simulink model "Lock_Control_Vy"  (Simulink 7.9)
settings: Solver=FixedStepDiscrete  StartTime=0.0  StopTime=0.8  RelTol=1e-3  SampleTimeConstraint=STIndependent
PreLoadFcn:
  | Locking_Strategy_selfinit
values from neighbouring files (symbols this model uses):
  lockDoor_speedThreshTimer = mpt.Parameter    [Locking_Strategy_selfinit.m]
  lockDoor_speedThreshValue = mpt.Parameter    [Locking_Strategy_selfinit.m]
libraries: common_lib x1
CloseFcn:
  | rtwprivate ssgencode ModelCloseRequest ADL
settings Model: MinMaxOverflowLogging=ForceOff  Creator=fguerin  LastModifiedBy=klindqvi  CovMetricSettings=dcme  CovHtmlReporting=off  covSaveCumulativeToWorkspaceVar=off  CovSaveSingleToWorkspaceVar=off  CovModelRefEnable=off  CovExternalEMLEnable=on
settings DataIOCC: ExternalInput=[t,u]  LimitDataPoints=off  LoadExternalInput=on  SaveOutput=off  DSMLogging=off  SaveTime=off  SignalLoggingName=logsOut
settings OptimizationCC: InlineParams=on  InlineInvariantSignals=on  EnhancedBackFolding=on  ZeroExternalMemoryAtStartup=off  ZeroInternalMemoryAtStartup=off  EfficientFloat2IntCast=on  OptimizeModelRefInitCode=on  LifeSpan=1
settings DebuggingCC: ReadBeforeWriteMsg=EnableAllAsError  WriteAfterWriteMsg=EnableAllAsError  WriteAfterReadMsg=EnableAllAsError  AlgebraicLoopMsg=error  ArtificialAlgebraicLoopMsg=error  SaveWithDisabledLinksMsg=error  SaveWithParameterizedLinksMsg=error  CheckExecutionContextPreStartOutputMsg=on  CheckExecutionContextRuntimeOutputMsg=on  BlockPriorityViolationMsg=error  SolverPrmCheckMsg=error  MultiTaskCondExecSysMsg=warning  MultiTaskRateTransMsg=warning  IntegerOverflowMsg=none  ParameterUnderflowMsg=error  ParameterPrecisionLossMsg=error  ParameterTunabilityLossMsg=error  UnderSpecifiedDataTypeMsg=warning  UnnecessaryDatatypeConvMsg=warning  VectorMatrixConversionMsg=error  SignalLabelMismatchMsg=warning  SFcnCompatibilityMsg=error  BusObjectLabelMismatch=error  RootOutportRequireBusObject=error  AssertControl=DisableAll  ModelReferenceIOMsg=error  ModelReferenceIOMismatchMessage=error  ModelReferenceCSMismatchMessage=warning  UnknownTsInhSupMsg=error  ModelReferenceDataLoggingMessage=error  ModelReferenceSymbolNameMessage=none  StrictBusMsg=ErrorOnBusTreatedAsVector
settings HardwareCC: ProdLargestAtomicInteger=Long  ProdLargestAtomicFloat=Double  ProdIntDivRoundTo=Zero  ProdEndianess=BigEndian  ProdHWDeviceType=Freescale->MPC5500
settings ModelReferenceCC: ModelReferenceNumInstancesAllowed=Single
settings SFSimCC: SimParseCustomCode=off
settings RTWCC: SystemTargetFile=ert.tlc  TemplateMakefile=ert_default_tmf  Description=Embedded Coder  GenerateReport=on  RTWVerbose=off  ProcessScript=ert_make_rtw_hook  IncludeHyperlinkInReport=on  LaunchReport=on  GenerateTraceInfo=on  GenerateTraceReport=on  GenerateTraceReportSl=on  GenerateTraceReportSf=on  GenerateTraceReportEml=on  GenerateCodeMetricsReport=on
settings MATStruct: className=rtw.pil.Bullseye  argsAllComponents=[]  excludedModels=[]  includeReferencedModels=off  includeTopModel=on  enabled=on
settings CodeAppCC: ForceParamTrailComments=on  IgnoreCustomStorageClasses=off  IgnoreTestpoints=on  MangleLength=4  InlinedPrmAccess=Macros  ReqsInCode=on
settings ERTTargetCC: CodeReplacementLibrary=ANSI_C  MultiwordLength=2048  SupportAbsoluteTime=off  SupportNonFinite=off  SupportComplex=off  PortableWordSizes=on  InlinedParameterPlacement=NonHierarchical  ERTCustomFileTemplate=example_file_process.tlc  ConvertIfToSwitch=off  SuppressUnreachableDefaultCases=off
settings ConfigComp: Description=Design Verifier Custom Configuration Component  DVMaxProcessTime=600  DVDisplayUnsatisfiableObjectives=on  DVAutomaticStubbing=off  DVOutputDir=C:\Work\Data\Pilots\P_PSA_ECoder_BenchMark_LaGarenne\source9b\deliverable\trunk\demos\VnV_example\Projects\ADL_Project/Simulink_Test_Generation/ADL_Sim  DVModelCoverageObjectives=MCDC  DVTestSuiteOptimization=CombinedObjectives  DVDataFileName=./Tests/$ModelName$_sldvdata  DVSaveHarnessModel=on  DVHarnessModelFileName=./Tests/$ModelName$_testHarness  DVModelReferenceHarness=on  DVSaveReport=on  DVReportFileName=ADL_Sim_SLDV.html

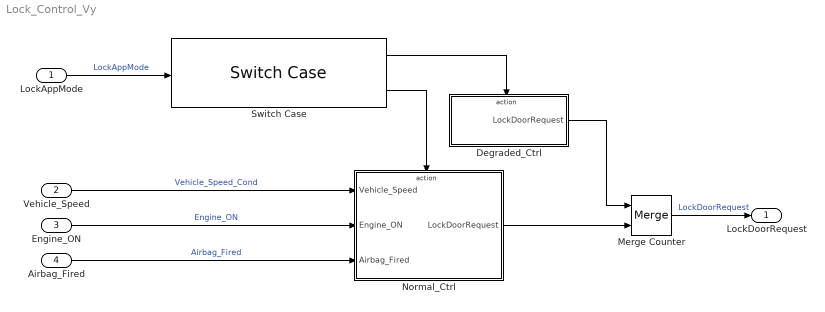
== system Lock_Control_Vy ==
  LockAppMode : Inport  PortDimensions=1
  Vehicle_Speed : Inport  Port=2  OutDataTypeStr=single  PortDimensions=1
  Engine_ON : Inport  Port=3  OutDataTypeStr=boolean  PortDimensions=1
  Airbag_Fired : Inport  Port=4  OutDataTypeStr=boolean  PortDimensions=1
  Degraded_Ctrl : Subsystem
  Merge Counter : Merge
  Normal_Ctrl : Subsystem
  Switch Case : SwitchCase  CaseConditions={LockingMode.FAILURE,[LockingMode.NORMAL_UNLOCK,LockingMode.NORMAL_LOCK]}  ShowDefaultCase=off
  LockDoorRequest : Outport  OutDataTypeStr=boolean  PortDimensions=1
  wires:
  LockAppMode/1 -> Switch Case/1  "LockAppMode"
  Vehicle_Speed/1 -> Normal_Ctrl/1(Vehicle_Speed)  "Vehicle_Speed_Cond"
  Engine_ON/1 -> Normal_Ctrl/2(Engine_ON)  "Engine_ON"
  Degraded_Ctrl/1(LockDoorRequest) -> Merge Counter/1
  Normal_Ctrl/1(LockDoorRequest) -> Merge Counter/2
  Merge Counter/1 -> LockDoorRequest/1  "LockDoorRequest"
  Switch Case/1 -> Degraded_Ctrl/Action
  Switch Case/2 -> Normal_Ctrl/Action
  Airbag_Fired/1 -> Normal_Ctrl/3(Airbag_Fired)  "Airbag_Fired"

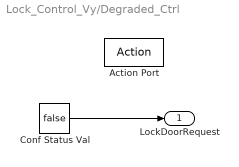
== system Lock_Control_Vy/Degraded_Ctrl ==
  Action Port : ActionPort  ActionType=case
  Conf Status Val : Constant  Value=false  OutDataTypeStr=Inherit: Inherit via back propagation  SampleTime=-1
  LockDoorRequest : Outport  OutDataTypeStr=boolean  PortDimensions=1
  wires:
  Conf Status Val/1 -> LockDoorRequest/1

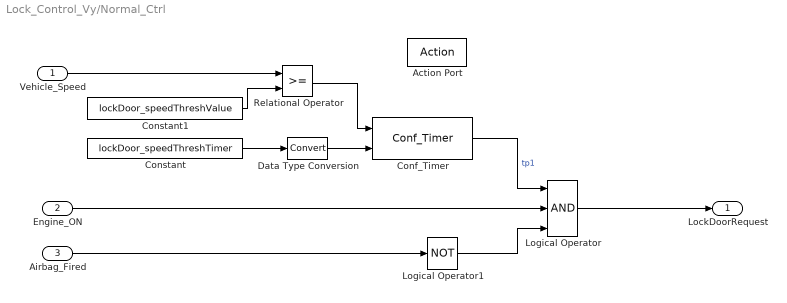
== system Lock_Control_Vy/Normal_Ctrl ==
  Vehicle_Speed : Inport  OutDataTypeStr=single  PortDimensions=1
  Engine_ON : Inport  Port=2  OutDataTypeStr=boolean  PortDimensions=1
  Airbag_Fired : Inport  Port=3  OutDataTypeStr=boolean  PortDimensions=1
  Action Port : ActionPort  ActionType=case
  Conf_Timer : common_lib/Conf_Timer
  Constant : Constant  RequirementInfo={}  Value=lockDoor_speedThreshTimer
  Constant1 : Constant  Value=lockDoor_speedThreshValue
  Data Type Conversion : DataTypeConversion  ConvertRealWorld=Stored Integer (SI)
  Logical Operator : Logic  Inputs=3  AllPortsSameDT=off  OutDataTypeStr=boolean
  Logical Operator1 : Logic  Operator=NOT  AllPortsSameDT=off  OutDataTypeStr=boolean
  Relational Operator : RelationalOperator  OutDataTypeStr=boolean
  LockDoorRequest : Outport  OutDataTypeStr=boolean  PortDimensions=1
  wires:
  Data Type Conversion/1 -> Conf_Timer/2
  Engine_ON/1 -> Logical Operator/2
  Logical Operator/1 -> LockDoorRequest/1
  Vehicle_Speed/1 -> Relational Operator/1
  Constant/1 -> Data Type Conversion/1
  Conf_Timer/1 -> Logical Operator/1  "tp1"
  Constant1/1 -> Relational Operator/2
  Relational Operator/1 -> Conf_Timer/1
  Airbag_Fired/1 -> Logical Operator1/1
  Logical Operator1/1 -> Logical Operator/3
